simulink model "driver_model_b_upd"  (R2023b)
settings: Solver=FixedStepDiscrete  StartTime=0  StopTime=45  FixedStep=0.0005  RelTol=1e-3  AbsTol=1e-6
InitFcn:
  | R2D = 180/pi;
libraries: Solver_SF x1, slpidlib x1
settings Model: DataTypeOverride=Double  MinMaxOverflowLogging=ForceOff  Creator=jhu  LastModifiedBy=rkddp
settings SolverCC: AutoScaleAbsTol=off  AlgebraicLoopSolver=TrustRegion
settings DataIOCC: SaveFormat=Array  ReturnWorkspaceOutputs=off  SignalLoggingName=sigsOut
settings OptimizationCC: BlockReduction=off  BooleanDataType=off  ExpressionDepthLimit=2147483647  InitFltsAndDblsToZero=on  LifeSpan=inf
settings DebuggingCC: SaveWithParameterizedLinksMsg=none  UnderspecifiedInitializationDetection=Classic  MergeDetectMultiDrivingBlocksExec=none  SignalResolutionControl=TryResolveAllWithWarning  MultiTaskDSMMsg=warning  MultiTaskCondExecSysMsg=none  ParameterPrecisionLossMsg=none  FcnCallInpInsideContextMsg=warning  UnconnectedInputMsg=warning  UnconnectedOutputMsg=warning  UnconnectedLineMsg=warning  StateNameClashWarn=warning  SFUnexpectedBacktrackingDiag=warning  SFNoUnconditionalDefaultTransitionDiag=warning  ArithmeticOperatorsInVariantConditions=warning
settings HardwareCC: ProdBitPerPointer=32  ProdBitPerSizeT=32  ProdBitPerPtrDiffT=32  ProdLargestAtomicFloat=None  ProdIntDivRoundTo=Undefined  ProdEndianess=Unspecified  ProdWordSize=32  ProdHWDeviceType=32-bit Generic  TargetHWDeviceType=32-bit Generic  TargetUnknown=on  ProdEqTarget=off
settings ModelReferenceCC: ModelReferenceMinAlgLoopOccurrences=on  PropagateSignalLabelsOutOfModel=off
settings SFSimCC: SimUseLocalCustomCode=off  CustomCodeUndefinedFunction=UseInterfaceOnly
settings RTWCC: TemplateMakefile=grt_vc.tmf  RTWUseLocalCustomCode=off
settings CodeAppCC: StateflowObjectComments=on
settings GRTTargetCC: TargetFcnLib=ansi_tfl_tmw.mat  TargetLangStandard=C89/C90 (ANSI)  CombineOutputUpdateFcns=off  GRTInterface=on
settings ConfigComp: CovMetricSettings=dw  CovSaveCumulativeToWorkspaceVar=on  CovSaveSingleToWorkspaceVar=on  CovExternalEMLEnable=off

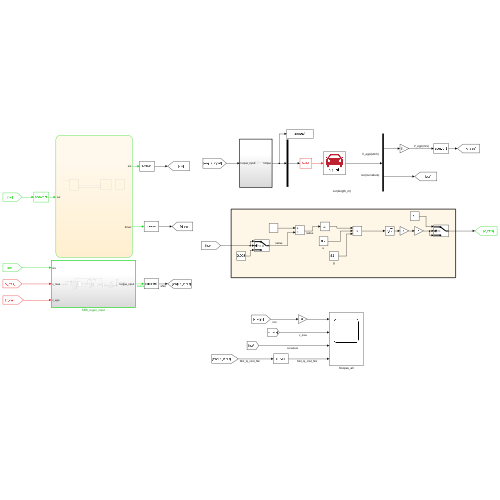
[thumbnail: Simulink's stored preview of the top-level diagram]
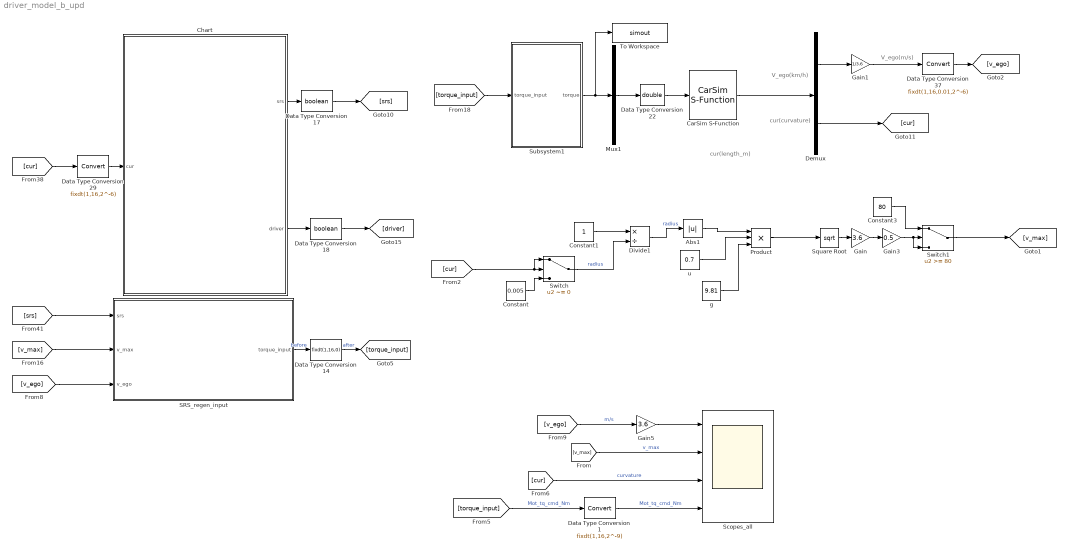
== system driver_model_b_upd ==
  note: V_ego(m/s)
  note: cur(curvature)
  note: V_ego(km/h)
  note: cur(length_m)
  Abs1 : Abs  SaturateOnIntegerOverflow=off
  CarSim S-Function : Solver_SF/CarSim S-Function  Priority=1  SIMFILE=simfile.sim  Run_RTs=off  vs_state_ind=Run  StopMode_ind=Vehicle Model
  Chart : Stateflow chart  TreatAsAtomicUnit=on  SystemSampleTime=0.01
  Constant : Constant  Value=0.005
  Constant1 : Constant
  Constant3 : Constant  Value=80
  Data Type Conversion1 : DataTypeConversion  OutDataTypeStr=fixdt(1,16,2^-9)  SaturateOnIntegerOverflow=off  RndMeth=Floor
  Data Type Conversion14 : DataTypeConversion  OutDataTypeStr=fixdt(1,16,0)  RndMeth=Nearest  SaturateOnIntegerOverflow=off
  Data Type Conversion17 : DataTypeConversion  OutDataTypeStr=boolean  SaturateOnIntegerOverflow=off  RndMeth=Floor
  Data Type Conversion18 : DataTypeConversion  OutDataTypeStr=boolean  SaturateOnIntegerOverflow=off  RndMeth=Floor
  Data Type Conversion22 : DataTypeConversion  OutDataTypeStr=double  RndMeth=Nearest  SaturateOnIntegerOverflow=off
  Data Type Conversion29 : DataTypeConversion  OutDataTypeStr=fixdt(1,16,2^-6)  RndMeth=Round  SaturateOnIntegerOverflow=off
  Data Type Conversion37 : DataTypeConversion  OutDataTypeStr=fixdt(1,16,0.01,2^-6)  RndMeth=Simplest  SaturateOnIntegerOverflow=off
  Demux : Demux  Outputs=2
  Divide1 : Product  Inputs=*/
  Gain : Gain  Gain=3.6
  Gain1 : Gain  Gain=1/3.6
  Gain3 : Gain  Gain=0.5
  Gain5 : Gain  Gain=3.6
  Mux1 : Mux  Inputs=1
  Product : Product  Inputs=3
  SRS_regen_input : Subsystem  TreatAsAtomicUnit=on  SystemSampleTime=0.01
  Scopes_all : Scope  NumInputPorts=4
  Square Root : Sqrt
  Subsystem1 : Subsystem  TreatAsAtomicUnit=on  SystemSampleTime=0.0005
  Switch : Switch  Criteria=u2 ~= 0  SaturateOnIntegerOverflow=off  InputSameDT=off
  Switch1 : Switch  Threshold=80  SaturateOnIntegerOverflow=off  InputSameDT=off
  To Workspace : ToWorkspace  VariableName=simout  SaveFormat=Timeseries  SampleTime=-1
  g : Constant  Value=9.81
  u : Constant  Value=0.7
  wires:
  Gain1/1 -> Data Type Conversion37/1
  [cur] -> Data Type Conversion29/1
  Chart/1(srs) -> Data Type Conversion17/1
  Chart/2(driver) -> Data Type Conversion18/1
  [srs] -> SRS_regen_input/1(srs)
  SRS_regen_input/1(torque_input) -> Data Type Conversion14/1  "before"
  [v_max] -> SRS_regen_input/2(v_max)
  CarSim S-Function/1 -> Demux/1
  Data Type Conversion37/1 -> [v_ego]
  Mux1/1 -> Data Type Conversion22/1
  Data Type Conversion14/1 -> [torque_input]  "after"
  Data Type Conversion17/1 -> [srs]
  Data Type Conversion18/1 -> [driver]
  Data Type Conversion22/1 -> CarSim S-Function/1
  Data Type Conversion29/1 -> Chart/1(cur)
  Demux/1 -> Gain1/1
  [v_ego] -> SRS_regen_input/3(v_ego)
  [torque_input] -> Subsystem1/1(torque_input)
  u/1 -> Product/2
  g/1 -> Product/3
  Product/1 -> Square Root/1
  Constant1/1 -> Divide1/1
  Divide1/1 -> Abs1/1  "radius"
  Subsystem1/1(torque) -> To Workspace/1, Mux1/1
  [cur] -> Switch/1, Switch/2
  Switch/1 -> Divide1/2  "radius"
  Constant/1 -> Switch/3
  Switch1/1 -> [v_max]
  Square Root/1 -> Gain/1
  Constant3/1 -> Switch1/1
  Data Type Conversion1/1 -> Scopes_all/4  "Mot_tq_cmd_Nm"
  [torque_input] -> Data Type Conversion1/1  "Mot_tq_cmd_Nm"
  [v_max] -> Scopes_all/2  "v_max"
  [v_ego] -> Gain5/1  "m/s"
  Demux/2 -> [cur]
  Abs1/1 -> Product/1
  Gain/1 -> Gain3/1
  Gain3/1 -> Switch1/3, Switch1/2
  [cur] -> Scopes_all/3  "curvature"
  Gain5/1 -> Scopes_all/1

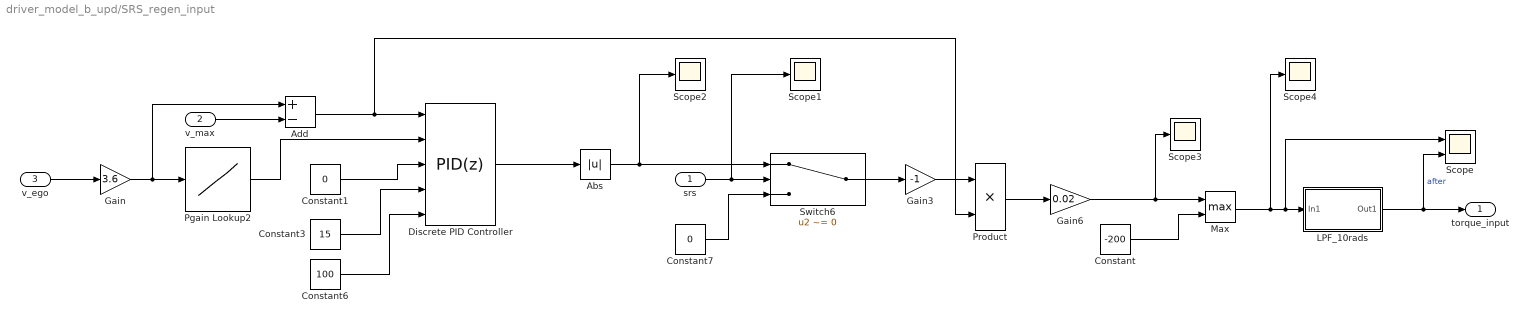
== system driver_model_b_upd/SRS_regen_input ==
  srs : Inport
  v_max : Inport  Port=2
  v_ego : Inport  Port=3
  Abs : Abs  SaturateOnIntegerOverflow=off
  Add : Sum  Inputs=+-
  Constant : Constant  Value=-200
  Constant1 : Constant  Value=0
  Constant3 : Constant  Value=15
  Constant6 : Constant  Value=100
  Constant7 : Constant  Value=0
  Discrete PID Controller : slpidlib/PID Controller  Controller=PID  Form=Parallel  TimeDomain=Discrete-time  UseExternalTs=off  SampleTime=0.01  IntegratorMethod=Forward Euler  FilterMethod=Forward Euler  ControllerParametersSource=external  P=1  I=1  UseKiTs=off  D=0  N=100  UseFilter=on  TunerSelectOption=Transfer Function Based (PID Tuner App)  InitialConditionSource=internal  InitialConditionForIntegrator=0  InitialConditionForFilter=0  DifferentiatorICPrevScaledInput=0  ExternalReset=none  TrackingMode=off  Kt=1  LimitOutput=off  SatLimitsSource=internal  UpperSaturationLimit=inf  LowerSaturationLimit=-inf  LinearizeAsGain=off  AntiWindupMode=none  Kb=1  LimitIntegrator=off  UpperIntegratorSaturationLimit=inf  LowerIntegratorSaturationLimit=-inf  POutMin=[]  POutMax=[]  IOutMin=[]  IOutMax=[]  DOutMin=[]  DOutMax=[]  NOutMin=[]  NOutMax=[]  SumOutMin=[]  SumOutMax=[]  SaturationOutMin=[]  SaturationOutMax=[]  PParamMin=[]  PParamMax=[]  IParamMin=[]  IParamMax=[]  DParamMin=[]  DParamMax=[]  NParamMin=[]  NParamMax=[]  KbParamMin=[]  KbParamMax=[]  KtParamMin=[]  KtParamMax=[]  KbOutMin=[]  KbOutMax=[]  KtOutMin=[]  KtOutMax=[]  IntegratorOutMin=[]  IntegratorOutMax=[]  FilterOutMin=[]  FilterOutMax=[]  SumI1OutMin=[]  SumI1OutMax=[]  SumI2OutMin=[]  SumI2OutMax=[]  SumI3OutMin=[]  SumI3OutMax=[]  SumI4OutMin=[]  SumI4OutMax=[]  SumDOutMin=[]  SumDOutMax=[]  DifferentiatorOutMin=[]  DifferentiatorOutMax=[]  FilterDiffOutCoefMin=[]  FilterDiffOutCoefMax=[]  ReciprocalOutMin=[]  ReciprocalOutMax=[]  SumDenOutMin=[]  SumDenOutMax=[]  SumNumOutMin=[]  SumNumOutMax=[]  DivideOutMin=[]  DivideOutMax=[]  UdiffTsProdOutMin=[]  UdiffTsProdOutMax=[]  NTsProdOutMin=[]  NTsProdOutMax=[]  UintegralTsProdOutMin=[]  UintegralTsProdOutMax=[]  UngainTsProdOutMin=[]  UngainTsProdOutMax=[]  ClampingZeroOutDataTypeStr=Inherit: Inherit via back propagation  ClampingZeroOutMin=[]  ClampingZeroOutMax=[]  FilterDenConstantOutDataTypeStr=Inherit: Inherit via back propagation  FilterDenConstantOutMin=[]  FilterDenConstantOutMax=[]  PCopyOutDataTypeStr=Inherit: Inherit via back propagation  PCopyOutMin=[]  PCopyOutMax=[]  NCopyOutDataTypeStr=Inherit: Inherit via back propagation  NCopyOutMin=[]  NCopyOutMax=[]  IntegratorContinuousStateAttributes=''  IntegratorStateMustResolveToSignalObject=off  IntegratorRTWStateStorageClass=Auto  FilterContinuousStateAttributes=''  FilterStateMustResolveToSignalObject=off  FilterRTWStateStorageClass=Auto  ParallelPVariant=ExternalParameters  IdealPVariant=Disabled  IVariant=ExternalParameters  DVariant=ExternalParameters  IntegratorVariant=Discrete  SatVariant=Disabled  AWVariant=Passthrough  PCopyVariant=Disabled  TRVariant=Disabled  FdbkBlocksVariant=Forward  IdealPFdbkVariant=Disabled  SatFdbkVariant=Disabled  DerivativeFilterVariant=ForwardEulerFilter  NVariant=ExternalParameters  NCopyVariant=Disabled  FilterICVariant=InternalICsFilter  IntegratorICVariant=InternalICs  ExternalResetVariant=Disabled  TRSumVariant=Passthrough  SumFdbkVariant=Disabled  SumVariant=Sum_PID  TsampFilterVariant=InternalTs  TsampNgainVariant=Passthrough  TsampIntegralVariant=Disabled_SignalSpec  ExternalSaturationOutDataTypeStr=Inherit: Same as second input
  Gain : Gain  Gain=3.6
  Gain3 : Gain  Gain=-1
  Gain6 : Gain  Gain=0.02
  LPF_10rads : Subsystem
  Max : MinMax  Function=max  Inputs=2
  Pgain Lookup2 : Lookup_n-D  NumberOfTableDimensions=1  BreakpointsForDimension1=[0 5 10 15 20 30 40 50 60 70 80 90 100 ]  Table=[45 45 50 50 50 50 50 50 50 55 55 55 55]  ExtrapMethod=Clip  UseLastTableValue=on  InternalRulePriority=Speed  RndMeth=Simplest
  Product : Product
  Scope : Scope  NumInputPorts=2
  Scope{1..4} (4 alike) : Scope
  Switch6 : Switch  Criteria=u2 ~= 0  SaturateOnIntegerOverflow=off  InputSameDT=off
  torque_input : Outport
  wires:
  Constant6/1 -> Discrete PID Controller/5
  Constant7/1 -> Switch6/3
  Constant3/1 -> Discrete PID Controller/4
  srs/1 -> Scope1/1, Switch6/2
  Abs/1 -> Scope2/1, Switch6/1
  Product/1 -> Gain6/1
  LPF_10rads/1(Out1) -> Scope/2, torque_input/1  "after"
  Constant1/1 -> Discrete PID Controller/3
  Gain3/1 -> Product/1
  Switch6/1 -> Gain3/1
  Gain6/1 -> Scope3/1, Max/1
  Constant/1 -> Max/2
  Pgain Lookup2/1 -> Discrete PID Controller/2
  Discrete PID Controller/1 -> Abs/1
  v_ego/1 -> Gain/1
  Max/1 -> Scope4/1, Scope/1, LPF_10rads/1(In1)
  Gain/1 -> Add/1, Pgain Lookup2/1
  v_max/1 -> Add/2
  Add/1 -> Product/2, Discrete PID Controller/1

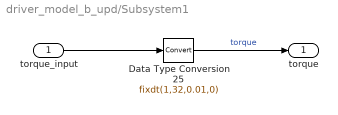
== system driver_model_b_upd/Subsystem1 ==
  torque_input : Inport
  Data Type Conversion25 : DataTypeConversion  OutDataTypeStr=fixdt(1,32,0.01,0)  SaturateOnIntegerOverflow=off  RndMeth=Floor
  torque : Outport
  wires:
  Data Type Conversion25/1 -> torque/1  "torque"
  torque_input/1 -> Data Type Conversion25/1

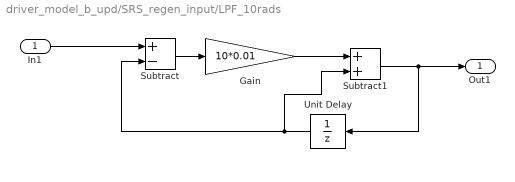
== system driver_model_b_upd/SRS_regen_input/LPF_10rads ==
  In1 : Inport
  Gain : Gain  Gain=10*0.01
  Subtract : Sum  Inputs=+-
  Subtract1 : Sum
  Unit Delay : UnitDelay  SampleTime=0.01  HasFrameUpgradeWarning=on
  Out1 : Outport
  wires:
  Subtract1/1 -> Out1/1, Unit Delay/1
  Unit Delay/1 -> Subtract/2, Subtract1/2
  Gain/1 -> Subtract1/1
  Subtract/1 -> Gain/1
  In1/1 -> Subtract/1

== stateflow chart driver_model_b_upd/Chart ==
  state INIT
    en:
    driver = 0;
    srs =0;
  state SRS_ON
    en:
    driver = 0;
    srs = 1;
  state Driver_ON
    en:
    driver = 1;
    srs = 0;
  (default) -> INIT
  INIT -> SRS_ON : [ cur > 0.002 || cur < -0.002 ]
  SRS_ON -> INIT : [cur == 0 || cur < 0.002 || cur > -0.002 || cur == 0.002 || cur == -0.002]
  data: srs output; driver output; cur input
